simulink model "modle_mavic"  (R2020b)
settings: Solver=VariableStepAuto  StartTime=0.0  StopTime=10.0  RelTol=1e-3
settings Model: Creator=boringtao  LastModifiedBy=boringtao

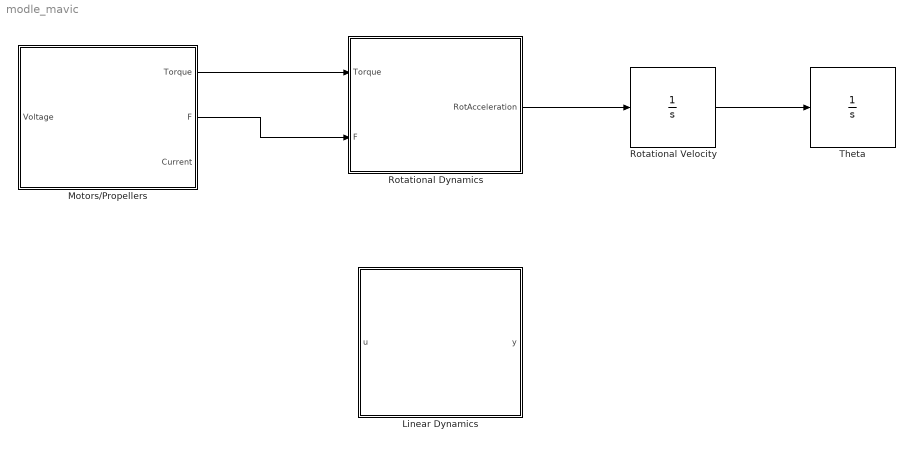
== system modle_mavic ==
  Linear Dynamics : MATLAB Function  TreatAsAtomicUnit=on
  Motors/Propellers : MATLAB Function  TreatAsAtomicUnit=on
  Rotational Dynamics : MATLAB Function  TreatAsAtomicUnit=on
  Rotational Velocity : Integrator
  Theta : Integrator
  wires:
  Motors/Propellers/1(Torque) -> Rotational Dynamics/1(Torque)
  Motors/Propellers/2(F) -> Rotational Dynamics/2(F)
  Rotational Dynamics/1(RotAcceleration) -> Rotational Velocity/1
  Rotational Velocity/1 -> Theta/1

== matlab function modle_mavic/Motors//Propellers ==
  data: Voltage input; Torque output; F output; Current output
function [Torque, F, Current] = fcn(Voltage)
RPM = [0 0 0 0]
Torque = [0 0 0 0]
Current = [0 0 0 0]
F = [0 0 0 0]

for i=1:4
    RPM(i) = -2.6932*Voltage(i)^3 + 1400*Voltage(i);
    Ct = 2*10^ - 15*RPM(i)^3 - 4*10^ - 11*RPM(i)^2 + 3*10^ - 7*RPM(i) + 0.1013;
    F(i) = Ct*1.225*(RPM(i)/60)^2*0.2^4;
    Torque(i) = 4*10^ -14*RPM(i)^3 + 8*10^ -12*RPM(i)^2 + 3*10^ -6*RPM(i);
    Current(i) = 1400*Torque(i);
end

== matlab function modle_mavic/Linear Dynamics ==
  data: u input; y output
function y = fcn(u)

y = u;

== matlab function modle_mavic/Rotational Dynamics ==
  data: Torque input; RotAcceleration output; F input
function RotAcceleration = fcn(Torque, F)
Moment = [0 0 0];
RotAcceleration = [0 0 0];
I = [0.003 0.003 0.007];

Moment(1) = (F(3) + F(4))*0.237/2 - (F(1) + F(2))*0.237/2
Moment(2) = (F(3) + F(2))*0.237/2 - (F(1) + F(4))*0.237/2
Moment(3) = Torque(4) - Torque(1) + Torque(2) - Torque(4)

for i = 1:3
    RotAcceleration(i) = Moment(i)/I(i);
end
